simulink library "nodeSpringDamperForce_ul"  (R2018b)
settings: Solver=VariableStepAuto  StartTime=0.0  StopTime=10.0  RelTol=1e-3
settings Model: Creator=mcobb  LastModifiedBy=mcobb

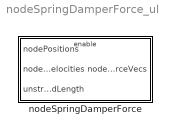
== system nodeSpringDamperForce_ul ==
  nodeSpringDamperForce : Subsystem  mask{mass=0, zeta=0, diameter=0, youngsMod=0}
      mask prompts: mass "Vehicle mass"; zeta "Tether damping ratio"; diameter "Tether diameter"; youngsMod "Youngs Modulus"

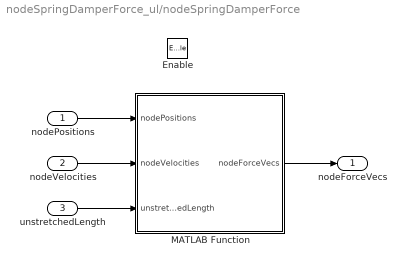
== system nodeSpringDamperForce_ul/nodeSpringDamperForce ==
  nodePositions : Inport
  nodeVelocities : Inport  Port=2
  unstretchedLength : Inport  Port=3
  Enable : EnablePort
  MATLAB Function : MATLAB Function  TreatAsAtomicUnit=on
  "nodeForceVecs " : Outport
  wires:
  nodePositions/1 -> MATLAB Function/1(nodePositions)
  nodeVelocities/1 -> MATLAB Function/2(nodeVelocities)
  MATLAB Function/1(nodeForceVecs) -> "nodeForceVecs "/1
  unstretchedLength/1 -> MATLAB Function/3(unstretchedLength)

== matlab function nodeSpringDamperForce_ul/nodeSpringDamperForce/MATLAB Function ==
  data: nodePositions input; nodeForceVecs output; nodeVelocities input; unstretchedLength input; mass parameter; zeta parameter; diameter parameter; youngsMod parameter
function nodeForceVecs = fcn(nodePositions,nodeVelocities,unstretchedLength,mass, zeta, diameter, youngsMod)

nodeForceVecs = nodeSpringDamperForce(nodePositions,nodeVelocities,unstretchedLength,mass,zeta,diameter,youngsMod);

end
